simulink model "Medium_Self_Balance_Vehicle"  (R2021b)
settings: Solver=FixedStepDiscrete  StartTime=0.0  StopTime=10.0  FixedStep=0.005  RelTol=1e-3
libraries: TIMERS_Lib x9, GPIO_Lib x8, REG_Lib x4, ADC_Lib x1, STM32_Config_Lib x1, USART_Lib x1
(part 1 of 2)
settings Model: Creator=Administrator  LastModifiedBy=Li Chong
settings SolverCC: AlgebraicLoopSolver=TrustRegion
settings DataIOCC: ReturnWorkspaceOutputs=off
settings OptimizationCC: DefaultParameterBehavior=Inlined  EnhancedBackFolding=on  PassReuseOutputArgsAs=Individual arguments  OptimizeBlockOrder=speed  DifferentSizesBufferReuse=on  OptimizationCustomize=off  EfficientTunableParamExpr=on
settings DebuggingCC: AlgebraicLoopMsg=none  MultiTaskDSMMsg=none  ParameterPrecisionLossMsg=none  ParameterTunabilityLossMsg=error  SFMachineParentedDataDiag=warning  ArithmeticOperatorsInVariantConditions=warning
settings HardwareCC: ProdBitPerPointer=32  ProdBitPerSizeT=32  ProdBitPerPtrDiffT=32  ProdLargestAtomicInteger=Integer  ProdWordSize=32  ProdHWDeviceType=STMicroelectronics->STM32 32-bit Cortex-M
settings SFSimCC: SimCustomHeaderCode="#include \"myfile.h\""  SimUserSources=myfile.c  SimUseLocalCustomCode=off  MATLABDynamicMemAlloc=off  CustomCodeUndefinedFunction=UseInterfaceOnly
settings RTWCC: Description=stm32 (Embedded Target)  SystemTargetFile=stm32.tlc  TemplateMakefile=stm32.tmf  GenerateReport=on  RTWUseLocalCustomCode=off  CustomHeaderCode="#include \"delay.h\""  IncludeHyperlinkInReport=on  GenerateTraceInfo=on  GenerateTraceReport=on  GenerateTraceReportSl=on  GenerateTraceReportSf=on  GenerateTraceReportEml=on
settings CodeAppCC: ForceParamTrailComments=on  IgnoreCustomStorageClasses=off  MaxIdLength=64  OperatorAnnotations=on  SimulinkDataObjDesc=on  SFDataObjDesc=on  CustomSymbolStrType=$N$R$M  SimulinkBlockComments=off
settings STFCustomTargetCC: TargetLangStandard=C99 (ISO)  CodeReplacementLibrary=ARM CMSIS SIN COS  MultiwordLength=256  ParMdlRefBuildCompliant=on  IncludeMdlTerminateFcn=off  CombineOutputUpdateFcns=on  ERTCustomFileBanners=on  SupportContinuousTime=off  SupportNonInlinedSFcns=off  RemoveResetFunc=on  MATLABClassNameForMDSCustomization=Simulink.SoftwareTarget.ERTCustomization  GRTInterface=off  SystemTargetFile=stm32.tlc
settings ERTTargetCC: TargetLangStandard=C99 (ISO)  CodeReplacementLibrary=ARM CMSIS SIN COS  CompOptLevelCompliant=off  ConcurrentExecutionCompliant=off  IncludeMdlTerminateFcn=off  ModelStepFunctionPrototypeControlCompliant=off  CPPClassGenCompliant=off  UseToolchainInfoCompliant=off  ExtModeStaticAllocSize=256  ExtModeMexArgs=0,1,115200,10  InlinedParameterPlacement=NonHierarchical  ERTSrcFileBannerTemplate=sourceFileTemplate.cgt  ERTHdrFileBannerTemplate=sourceFileTemplate.cgt  ERTDataSrcFileTemplate=sourceFileTemplate.cgt  ERTDataHdrFileTemplate=sourceFileTemplate.cgt  ERTCustomFileTemplate=customRoutineProcess.tlc

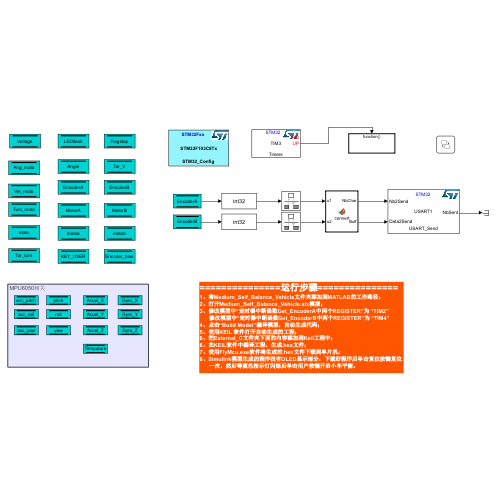
[thumbnail: Simulink's stored preview of the top-level diagram]
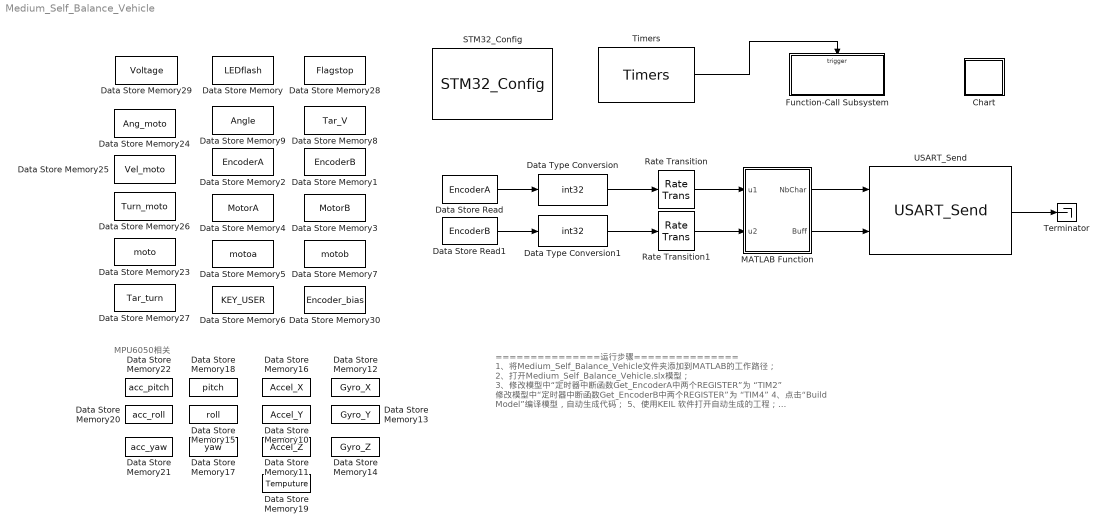
== system Medium_Self_Balance_Vehicle ==
  note: MPU6050相关
  note: ===============运行步骤===============
      | 1、将Medium_Self_Balance_Vehicle文件夹添加到MATLAB的工作路径；
      | 2、打开Medium_Self_Balance_Vehicle.slx模型；
      | 3、修改模型中“定时器中断函数Get_EncoderA中两个REGISTER”为 “TIM2”
      | 修改模型中“定时器中断函数Get_EncoderB中两个REGISTER”为 “TIM4”
      | 4、点击“Build Model”编译模型，自动生成代码；
      | 5、使用KEIL 软件打开自动生成的工程；
      | 6、把External_C文件夹下面的内容添加到Keil工程中；
      | 6、在KEIL软件中编译工程，生成.hex文件；
      | 7、使用FlyMcu.exe软件将生成的.hex文件下载到单片机；
      | 8、Simulink模型生成的程序没有OLED显示部分，下载好程序后单击复位按键复位 一次，然后等蓝色指示灯闪烁后单击用户按键开启小车平衡。
  Chart : Stateflow chart  Priority=1  TreatAsAtomicUnit=on
  Data Store Memory : DataStoreMemory  DataStoreName=LEDflash  ReadBeforeWriteMsg=warning  WriteAfterWriteMsg=warning  WriteAfterReadMsg=warning  ShowAdditionalParam=off
  Data Store Memory1 : DataStoreMemory  DataStoreName=EncoderB  ReadBeforeWriteMsg=warning  WriteAfterWriteMsg=warning  WriteAfterReadMsg=warning  ShowAdditionalParam=off  OutDataTypeStr=int16
  Data Store Memory10 : DataStoreMemory  DataStoreName=Accel_Y  ReadBeforeWriteMsg=warning  WriteAfterWriteMsg=warning  WriteAfterReadMsg=warning  ShowAdditionalParam=off  OutDataTypeStr=double
  Data Store Memory11 : DataStoreMemory  DataStoreName=Accel_Z  ReadBeforeWriteMsg=warning  WriteAfterWriteMsg=warning  WriteAfterReadMsg=warning  ShowAdditionalParam=off  OutDataTypeStr=double
  Data Store Memory12 : DataStoreMemory  DataStoreName=Gyro_X  ReadBeforeWriteMsg=warning  WriteAfterWriteMsg=warning  WriteAfterReadMsg=warning  ShowAdditionalParam=off  OutDataTypeStr=double
  Data Store Memory13 : DataStoreMemory  DataStoreName=Gyro_Y  ReadBeforeWriteMsg=warning  WriteAfterWriteMsg=warning  WriteAfterReadMsg=warning  ShowAdditionalParam=off  OutDataTypeStr=double
  Data Store Memory14 : DataStoreMemory  DataStoreName=Gyro_Z  ReadBeforeWriteMsg=warning  WriteAfterWriteMsg=warning  WriteAfterReadMsg=warning  ShowAdditionalParam=off  OutDataTypeStr=double
  Data Store Memory15 : DataStoreMemory  DataStoreName=roll  ReadBeforeWriteMsg=warning  WriteAfterWriteMsg=warning  WriteAfterReadMsg=warning  ShowAdditionalParam=off  OutDataTypeStr=double
  Data Store Memory16 : DataStoreMemory  DataStoreName=Accel_X  ReadBeforeWriteMsg=warning  WriteAfterWriteMsg=warning  WriteAfterReadMsg=warning  ShowAdditionalParam=off  OutDataTypeStr=double
  Data Store Memory17 : DataStoreMemory  DataStoreName=yaw  ReadBeforeWriteMsg=warning  WriteAfterWriteMsg=warning  WriteAfterReadMsg=warning  ShowAdditionalParam=off  OutDataTypeStr=double
  Data Store Memory18 : DataStoreMemory  DataStoreName=pitch  ReadBeforeWriteMsg=warning  WriteAfterWriteMsg=warning  WriteAfterReadMsg=warning  ShowAdditionalParam=off  OutDataTypeStr=double
  Data Store Memory19 : DataStoreMemory  DataStoreName=Temputure  ReadBeforeWriteMsg=warning  WriteAfterWriteMsg=warning  WriteAfterReadMsg=warning  ShowAdditionalParam=off  OutDataTypeStr=double
  Data Store Memory2 : DataStoreMemory  DataStoreName=EncoderA  ReadBeforeWriteMsg=warning  WriteAfterWriteMsg=warning  WriteAfterReadMsg=warning  ShowAdditionalParam=off  OutDataTypeStr=int16
  Data Store Memory20 : DataStoreMemory  DataStoreName=acc_roll  ReadBeforeWriteMsg=warning  WriteAfterWriteMsg=warning  WriteAfterReadMsg=warning  ShowAdditionalParam=off  OutDataTypeStr=double
  Data Store Memory21 : DataStoreMemory  DataStoreName=acc_yaw  ReadBeforeWriteMsg=warning  WriteAfterWriteMsg=warning  WriteAfterReadMsg=warning  ShowAdditionalParam=off  OutDataTypeStr=double
  Data Store Memory22 : DataStoreMemory  DataStoreName=acc_pitch  ReadBeforeWriteMsg=warning  WriteAfterWriteMsg=warning  WriteAfterReadMsg=warning  ShowAdditionalParam=off  OutDataTypeStr=double
  Data Store Memory23 : DataStoreMemory  DataStoreName=moto  ReadBeforeWriteMsg=warning  WriteAfterWriteMsg=warning  WriteAfterReadMsg=warning  ShowAdditionalParam=off
  Data Store Memory24 : DataStoreMemory  DataStoreName=Ang_moto  ReadBeforeWriteMsg=warning  WriteAfterWriteMsg=warning  WriteAfterReadMsg=warning  ShowAdditionalParam=off
  Data Store Memory25 : DataStoreMemory  DataStoreName=Vel_moto  ReadBeforeWriteMsg=warning  WriteAfterWriteMsg=warning  WriteAfterReadMsg=warning  ShowAdditionalParam=off
  Data Store Memory26 : DataStoreMemory  DataStoreName=Turn_moto  ReadBeforeWriteMsg=warning  WriteAfterWriteMsg=warning  WriteAfterReadMsg=warning  ShowAdditionalParam=off
  Data Store Memory27 : DataStoreMemory  DataStoreName=Tar_turn  ReadBeforeWriteMsg=warning  WriteAfterWriteMsg=warning  WriteAfterReadMsg=warning  ShowAdditionalParam=off
  Data Store Memory28 : DataStoreMemory  DataStoreName=Flagstop  ReadBeforeWriteMsg=warning  WriteAfterWriteMsg=warning  WriteAfterReadMsg=warning  InitialValue=1  ShowAdditionalParam=off  OutDataTypeStr=boolean
  Data Store Memory29 : DataStoreMemory  DataStoreName=Voltage  ReadBeforeWriteMsg=warning  WriteAfterWriteMsg=warning  WriteAfterReadMsg=warning  ShowAdditionalParam=off  OutDataTypeStr=double
  Data Store Memory3 : DataStoreMemory  DataStoreName=MotorB  ReadBeforeWriteMsg=warning  WriteAfterWriteMsg=warning  WriteAfterReadMsg=warning  ShowAdditionalParam=off  OutDataTypeStr=double
  Data Store Memory30 : DataStoreMemory  DataStoreName=Encoder_bias  ReadBeforeWriteMsg=warning  WriteAfterWriteMsg=warning  WriteAfterReadMsg=warning  ShowAdditionalParam=off  OutDataTypeStr=double
  Data Store Memory4 : DataStoreMemory  DataStoreName=MotorA  ReadBeforeWriteMsg=warning  WriteAfterWriteMsg=warning  WriteAfterReadMsg=warning  ShowAdditionalParam=off  OutDataTypeStr=double
  Data Store Memory5 : DataStoreMemory  DataStoreName=motoa  ReadBeforeWriteMsg=warning  WriteAfterWriteMsg=warning  WriteAfterReadMsg=warning  ShowAdditionalParam=off  OutDataTypeStr=int16
  Data Store Memory6 : DataStoreMemory  DataStoreName=KEY_USER  ReadBeforeWriteMsg=warning  WriteAfterWriteMsg=warning  WriteAfterReadMsg=warning  ShowAdditionalParam=off  OutDataTypeStr=int16
  Data Store Memory7 : DataStoreMemory  DataStoreName=motob  ReadBeforeWriteMsg=warning  WriteAfterWriteMsg=warning  WriteAfterReadMsg=warning  ShowAdditionalParam=off  OutDataTypeStr=int16
  Data Store Memory8 : DataStoreMemory  DataStoreName=Tar_V  ReadBeforeWriteMsg=warning  WriteAfterWriteMsg=warning  WriteAfterReadMsg=warning  ShowAdditionalParam=off  OutDataTypeStr=int16
  Data Store Memory9 : DataStoreMemory  DataStoreName=Angle  ReadBeforeWriteMsg=warning  WriteAfterWriteMsg=warning  WriteAfterReadMsg=warning  ShowAdditionalParam=off  OutDataTypeStr=double
  Data Store Read : DataStoreRead  DataStoreName=EncoderA  SampleTime=0.05  IndexOptions=Index vector (dialog)  Indices=1  OutputSizes=1
  Data Store Read1 : DataStoreRead  DataStoreName=EncoderB  SampleTime=0.05  IndexOptions=Index vector (dialog)  Indices=1  OutputSizes=1
  Data Type Conversion : DataTypeConversion  OutDataTypeStr=int32
  Data Type Conversion1 : DataTypeConversion  OutDataTypeStr=int32
  Function-Call Subsystem : Subsystem  TreatAsAtomicUnit=on
  MATLAB Function : MATLAB Function  TreatAsAtomicUnit=on
  Rate Transition : RateTransition  OutPortSampleTimeMultiple=10  OutPortSampleTime=0.05
  Rate Transition1 : RateTransition  OutPortSampleTimeMultiple=10  OutPortSampleTime=0.05
  STM32_Config : STM32_Config_Lib/STM32_Config  Priority=0  Project_Path=.\  Config_File=Medium_Self_Balance_Vehicle.ioc  MCU_Name=STM32F103C8Tx
      settings: SourceProductName=Target Support Package - STM32 Adapter
  Terminator : Terminator
  Timers : TIMERS_Lib/Timers  Priority=2  currentTIM=TIM3  TIM_Name=TIM3  sysUsingTimer=off  TIM_APBClock=72000000  TIM_Set_Clk=off  TIM_Prescaler=7199  TIM_Clock=10000.00  Variable_frequency=off  TIM_Set_OutFreq=off  TIM_ARR=49  Output_frequency=204.08  Repetition_counter=0  TIM_Mode=Up  TIM_DMA=none  TIM_IRQ=on  TIM_IRQ_ONLY=on  TIM_UP=on  TIM_TRG=off  TIM_COM=off  TIM_BRK=off  NbTIM=4  CH1_enable=off  CH1N_enable=off  CH1_type=Unknown  CH1_DMA=off  CH1_int=off  CH1_edge=Rising  CH1_div=1  CH1_variable_duty=off  CH1_set_pulse=off  CH1_output_duty=0.00  CH1_pulse=0  CH2_enable=off  CH2N_enable=off  CH2_type=Unknown  CH2_DMA=off  CH2_int=off  CH2_edge=Rising  CH2_div=1  CH2_variable_duty=off  CH2_set_pulse=off  CH2_output_duty=0.00  CH2_pulse=0  CH3_enable=off  CH3N_enable=off  CH3_type=Unknown  CH3_DMA=off  CH3_int=off  CH3_edge=Rising  CH3_div=1  CH3_variable_duty=off  CH3_set_pulse=off  CH3_output_duty=0.00  CH3_pulse=0  CH4_enable=off  CH4N_enable=off  CH4_type=Unknown  CH4_DMA=off  CH4_int=off  CH4_edge=Rising  CH4_div=1  CH4_variable_duty=off  CH4_set_pulse=off  CH4_output_duty=0.00  CH4_pulse=0
      settings: SourceProductName=Target Support Package - STM32 Adapter
  USART_Send : USART_Lib/USART_Send  USART_name=USART1  Buff_size=56  nbUsart=1  usartMode=Asynchronous  usartDma_Rx=off  usartDma_Tx=off  usartIt=on
      settings: SourceProductName=Target Support Package - STM32 Adapter
  wires:
  MATLAB Function/1(NbChar) -> USART_Send/1
  Data Store Read/1 -> Data Type Conversion/1
  USART_Send/1 -> Terminator/1
  MATLAB Function/2(Buff) -> USART_Send/2
  Data Store Read1/1 -> Data Type Conversion1/1
  Timers/1 -> Function-Call Subsystem/Trigger
  Data Type Conversion1/1 -> Rate Transition1/1
  Data Type Conversion/1 -> Rate Transition/1
  Rate Transition1/1 -> MATLAB Function/2(u2)
  Rate Transition/1 -> MATLAB Function/1(u1)

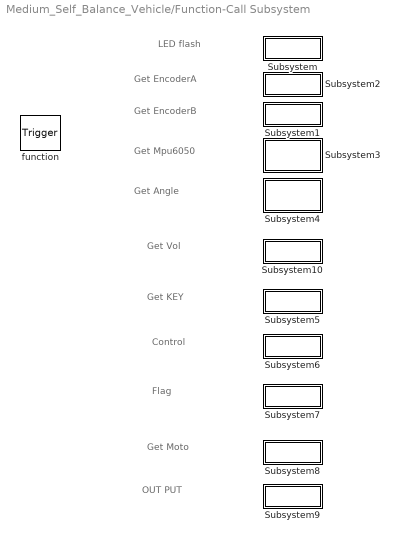
== system Medium_Self_Balance_Vehicle/Function-Call Subsystem ==
  note: Get Moto
  note: Get EncoderA
  note: OUT PUT
  note: LED flash
  note: Get KEY
  note: Get EncoderB
  note: Get Mpu6050
  note: Get Angle
  note: Control
  note: Flag
  note: Get Vol
  function : TriggerPort  TriggerType=function-call  VariantControl=Variant
  Subsystem : Subsystem  Priority=0
  Subsystem1 : Subsystem  Priority=1
  Subsystem10 : Subsystem  Priority=4
  Subsystem2 : Subsystem  Priority=1
  Subsystem3 : Subsystem  Priority=2
  Subsystem4 : Subsystem  Priority=3
  Subsystem5 : Subsystem  Priority=5
  Subsystem6 : Subsystem  Priority=6
  Subsystem7 : Subsystem  Priority=7
  Subsystem8 : Subsystem  Priority=8
  Subsystem9 : Subsystem  Priority=9

== system Medium_Self_Balance_Vehicle/Function-Call Subsystem/Subsystem ==
  Add : Sum
  Constant : Constant
  Data Store Read1 : DataStoreRead  DataStoreName=LEDflash  IndexOptions=Index vector (dialog)  Indices=1  OutputSizes=1
  Data Store Write : DataStoreWrite  DataStoreName=LEDflash  IndexOptions=Index vector (dialog)  Indices=1  OutputSizes=1
  If : If  IfExpression=u1 > 200
  If Action Subsystem : Subsystem  TreatAsAtomicUnit=on
  Terminator : Terminator
  wires:
  Constant/1 -> Add/2
  If/1 -> If Action Subsystem/Action
  If/2 -> Terminator/1
  Add/1 -> Data Store Write/1, If/1
  Data Store Read1/1 -> Add/1

== system Medium_Self_Balance_Vehicle/Function-Call Subsystem/Subsystem1 ==
  Data Store Write1 : DataStoreWrite  Priority=2  DataStoreName=EncoderB  IndexOptions=Index vector (dialog)  Indices=1  OutputSizes=1
  REG_Access2 : REG_Lib/REG_Access  Priority=2  Peripheral=ADC1  RegName=CNT  RegRead=off  RegWrite=on  RegValueIn=off  RegValue=0  RegEqual=on  RegAnd=off  RegOr=off  RegComplement=off  currentPeriph=ADC1
      settings: SourceProductName=Target Support Package - STM32 Adapter
  REG_Access3 : REG_Lib/REG_Access  Priority=1  Peripheral=ADC1  RegName=CNT  RegRead=on  RegWrite=off  RegValueIn=off  RegValue=0  RegEqual=on  RegAnd=off  RegOr=off  RegComplement=off  currentPeriph=ADC1
      settings: SourceProductName=Target Support Package - STM32 Adapter
  Timers1 : TIMERS_Lib/Timers  currentTIM=TIM4  TIM_Name=TIM4  sysUsingTimer=off  TIM_APBClock=72000000  TIM_Set_Clk=off  TIM_Prescaler=0  TIM_Clock=72000000.00  Variable_frequency=off  TIM_Set_OutFreq=off  TIM_ARR=65536  Output_frequency=1098.63  Repetition_counter=0  TIM_Mode=Up  TIM_DMA=none  TIM_IRQ=on  TIM_IRQ_ONLY=on  TIM_UP=off  TIM_TRG=off  TIM_COM=off  TIM_BRK=off  NbTIM=4  CH1_enable=on  CH1N_enable=off  CH1_type=Input_Encoder  CH1_DMA=off  CH1_int=off  CH1_edge=Rising  CH1_div=1  CH1_variable_duty=off  CH1_set_pulse=off  CH1_output_duty=0.00  CH1_pulse=0  CH2_enable=on  CH2N_enable=off  CH2_type=Input_Encoder  CH2_DMA=off  CH2_int=off  CH2_edge=Rising  CH2_div=1  CH2_variable_duty=off  CH2_set_pulse=off  CH2_output_duty=0.00  CH2_pulse=0  CH3_enable=off  CH3N_enable=off  CH3_type=Unknown  CH3_DMA=off  CH3_int=off  CH3_edge=Rising  CH3_div=1  CH3_variable_duty=off  CH3_set_pulse=off  CH3_output_duty=0.00  CH3_pulse=0  CH4_enable=off  CH4N_enable=off  CH4_type=Unknown  CH4_DMA=off  CH4_int=off  CH4_edge=Rising  CH4_div=1  CH4_variable_duty=off  CH4_set_pulse=off  CH4_output_duty=0.00  CH4_pulse=0
      settings: SourceProductName=Target Support Package - STM32 Adapter
  wires:
  REG_Access3/1 -> Data Store Write1/1

== system Medium_Self_Balance_Vehicle/Function-Call Subsystem/Subsystem10 ==
  1/10 : Gain  Gain=0.1
  3.3*11/4096 : Gain  Gain=0.00886
  ADC_Read : ADC_Lib/ADC_Read  Priority=1  ADC_Name=ADC1  ADC_Ch0=off  ADC_Ch1=off  ADC_Ch2=off  ADC_Ch3=off  ADC_Ch4=off  ADC_Ch5=off  ADC_Ch6=on  ADC_Ch7=off  ADC_Ch8=off  ADC_Ch9=off  ADC_Ch10=off  ADC_Ch11=off  ADC_Ch12=off  ADC_Ch13=off  ADC_Ch14=off  ADC_Ch15=off  ADC_Ch16=off  ADC_Ch17=off  ADC_Ch18=off  RgRk1=on  RgRk2=off  RgRk3=off  RgRk4=off  RgRk1_Ch=Ch6_r1  RgRk2_Ch=off  RgRk3_Ch=off  RgRk4_Ch=off  RgRk5=off  RgRk6=off  RgRk7=off  RgRk8=off  RgRk5_Ch=off  RgRk6_Ch=off  RgRk7_Ch=off  RgRk8_Ch=off  RgRk9=off  RgRk10=off  RgRk11=off  RgRk12=off  RgRk9_Ch=off  RgRk10_Ch=off  RgRk11_Ch=off  RgRk12_Ch=off  RgRk13=off  RgRk14=off  RgRk15=off  RgRk16=off  RgRk13_Ch=off  RgRk14_Ch=off  RgRk15_Ch=off  RgRk16_Ch=off  InjRk1=off  InjRk2=off  InjRk3=off  InjRk4=off  InjRk1_Ch=off  InjRk2_Ch=off  InjRk3_Ch=off  InjRk4_Ch=off  ADC_Trig=Not used  ADC_TrigEdge=Not used  DmaReq=off  DMA_Buffer=0  ItReq=off  AWD_Mode=NOT_USED  AWD_Ch=0  AWD_HThres=0  AWD_LThres=0  AWD_En_Int=off  AWD2_HThres=0  AWD2_LThres=0  AWD2_En_Int=off  AWD3_HThres=0  AWD3_LThres=0  AWD3_En_Int=off  EOC_SEQ=off  EOC_IT=off  JEOC_IT=off  AWD_IT=off  OVR_IT=off  CpltTrans=off  HalfTrans=off  ADC_RegNb=1  ADC_RegCh0=off  ADC_RegCh1=off  ADC_RegCh2=off  ADC_RegCh3=off  ADC_RegCh4=off  ADC_RegCh5=off  ADC_RegCh6=on  ADC_RegCh7=off  ADC_RegCh8=off  ADC_RegCh9=off  ADC_RegCh10=off  ADC_RegCh11=off  ADC_RegCh12=off  ADC_RegCh13=off  ADC_RegCh14=off  ADC_RegCh15=off  ADC_RegCh16=off  ADC_RegCh17=off  ADC_RegCh18=off  ADC_InjNb=0  ADC_InjCh0=off  ADC_InjCh1=off  ADC_InjCh2=off  ADC_InjCh3=off  ADC_InjCh4=off  ADC_InjCh5=off  ADC_InjCh6=off  ADC_InjCh7=off  ADC_InjCh8=off  ADC_InjCh9=off  ADC_InjCh10=off  ADC_InjCh11=off  ADC_InjCh12=off  ADC_InjCh13=off  ADC_InjCh14=off  ADC_InjCh15=off  ADC_InjCh16=off  ADC_InjCh17=off  ADC_InjCh18=off  NbADC=1  CurrentADC=ADC1
      settings: SourceProductName=Target Support Package - STM32 Adapter
  Data Store Write : DataStoreWrite  DataStoreName=Voltage  IndexOptions=Index vector (dialog)  Indices=1  OutputSizes=1
  For Iterator Subsystem1 : Subsystem  Priority=4  TreatAsAtomicUnit=on
  wires:
  For Iterator Subsystem1/1(Out1) -> 1/10/1
  1/10/1 -> 3.3*11/4096/1
  3.3*11/4096/1 -> Data Store Write/1
  ADC_Read/1 -> For Iterator Subsystem1/1(In1)

== system Medium_Self_Balance_Vehicle/Function-Call Subsystem/Subsystem2 ==
  Data Store Write4 : DataStoreWrite  Priority=2  DataStoreName=EncoderA  IndexOptions=Index vector (dialog)  Indices=1  OutputSizes=1
  REG_Access : REG_Lib/REG_Access  Priority=2  Peripheral=ADC1  RegName=CNT  RegRead=off  RegWrite=on  RegValueIn=off  RegValue=0  RegEqual=on  RegAnd=off  RegOr=off  RegComplement=off  currentPeriph=ADC1
      settings: SourceProductName=Target Support Package - STM32 Adapter
  REG_Access1 : REG_Lib/REG_Access  Priority=1  Peripheral=ADC1  RegName=CNT  RegRead=on  RegWrite=off  RegValueIn=off  RegValue=0  RegEqual=on  RegAnd=off  RegOr=off  RegComplement=off  currentPeriph=ADC1
      settings: SourceProductName=Target Support Package - STM32 Adapter
  Timers : TIMERS_Lib/Timers  currentTIM=TIM2  TIM_Name=TIM2  sysUsingTimer=off  TIM_APBClock=72000000  TIM_Set_Clk=off  TIM_Prescaler=0  TIM_Clock=72000000.00  Variable_frequency=off  TIM_Set_OutFreq=off  TIM_ARR=65536  Output_frequency=1098.63  Repetition_counter=0  TIM_Mode=Up  TIM_DMA=none  TIM_IRQ=on  TIM_IRQ_ONLY=on  TIM_UP=off  TIM_TRG=off  TIM_COM=off  TIM_BRK=off  NbTIM=4  CH1_enable=on  CH1N_enable=off  CH1_type=Input_Encoder  CH1_DMA=off  CH1_int=off  CH1_edge=Rising  CH1_div=1  CH1_variable_duty=off  CH1_set_pulse=off  CH1_output_duty=0.00  CH1_pulse=0  CH2_enable=on  CH2N_enable=off  CH2_type=Input_Encoder  CH2_DMA=off  CH2_int=off  CH2_edge=Rising  CH2_div=1  CH2_variable_duty=off  CH2_set_pulse=off  CH2_output_duty=0.00  CH2_pulse=0  CH3_enable=off  CH3N_enable=off  CH3_type=Unknown  CH3_DMA=off  CH3_int=off  CH3_edge=Rising  CH3_div=1  CH3_variable_duty=off  CH3_set_pulse=off  CH3_output_duty=0.00  CH3_pulse=0  CH4_enable=off  CH4N_enable=off  CH4_type=Unknown  CH4_DMA=off  CH4_int=off  CH4_edge=Rising  CH4_div=1  CH4_variable_duty=off  CH4_set_pulse=off  CH4_output_duty=0.00  CH4_pulse=0
      settings: SourceProductName=Target Support Package - STM32 Adapter
  wires:
  REG_Access1/1 -> Data Store Write4/1

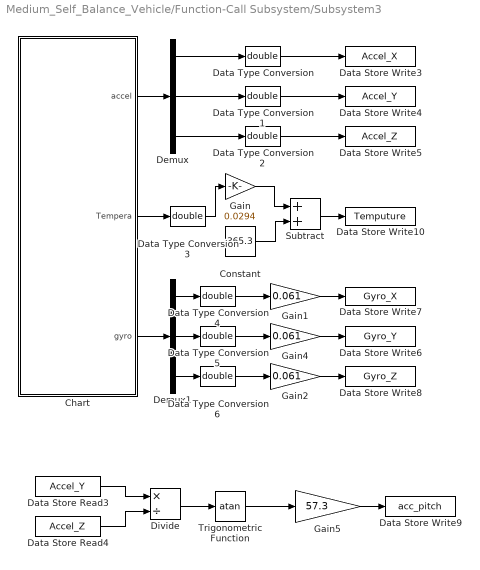
== system Medium_Self_Balance_Vehicle/Function-Call Subsystem/Subsystem3 ==
  Chart : Stateflow chart  TreatAsAtomicUnit=on
  Constant : Constant  Value=365.3  OutDataTypeStr=double
  Data Store Read3 : DataStoreRead  DataStoreName=Accel_Y  IndexOptions=Index vector (dialog)  Indices=1  OutputSizes=1
  Data Store Read4 : DataStoreRead  DataStoreName=Accel_Z  IndexOptions=Index vector (dialog)  Indices=1  OutputSizes=1
  Data Store Write10 : DataStoreWrite  DataStoreName=Temputure  IndexOptions=Index vector (dialog)  Indices=1  OutputSizes=1
  Data Store Write3 : DataStoreWrite  DataStoreName=Accel_X  IndexOptions=Index vector (dialog)  Indices=1  OutputSizes=1
  Data Store Write4 : DataStoreWrite  DataStoreName=Accel_Y  IndexOptions=Index vector (dialog)  Indices=1  OutputSizes=1
  Data Store Write5 : DataStoreWrite  DataStoreName=Accel_Z  IndexOptions=Index vector (dialog)  Indices=1  OutputSizes=1
  Data Store Write6 : DataStoreWrite  DataStoreName=Gyro_Y  IndexOptions=Index vector (dialog)  Indices=1  OutputSizes=1
  Data Store Write7 : DataStoreWrite  DataStoreName=Gyro_X  IndexOptions=Index vector (dialog)  Indices=1  OutputSizes=1
  Data Store Write8 : DataStoreWrite  DataStoreName=Gyro_Z  IndexOptions=Index vector (dialog)  Indices=1  OutputSizes=1
  Data Store Write9 : DataStoreWrite  DataStoreName=acc_pitch  IndexOptions=Index vector (dialog)  Indices=1  OutputSizes=1
  Data Type Conversion{,1..6} (7 alike) : DataTypeConversion  OutDataTypeStr=double
  Demux : Demux  Outputs=3
  Demux1 : Demux  Outputs=3
  Divide : Product  Inputs=*/
  Gain : Gain  Gain=0.0294  OutDataTypeStr=double
  Gain1 : Gain  Gain=0.061  OutDataTypeStr=double
  Gain2 : Gain  Gain=0.061  OutDataTypeStr=double
  Gain4 : Gain  Gain=0.061  OutDataTypeStr=double
  Gain5 : Gain  Gain=57.3  OutDataTypeStr=double
  Subtract : Sum  OutDataTypeStr=double
  Trigonometric Function : Trigonometry  Operator=atan
  wires:
  Demux/2 -> Data Type Conversion1/1
  Demux/1 -> Data Type Conversion/1
  Demux/3 -> Data Type Conversion2/1
  Demux1/2 -> Data Type Conversion5/1
  Demux1/3 -> Data Type Conversion6/1
  Demux1/1 -> Data Type Conversion4/1
  Chart/3(gyro) -> Demux1/1
  Chart/1(accel) -> Demux/1
  Gain/1 -> Subtract/1
  Constant/1 -> Subtract/2
  Subtract/1 -> Data Store Write10/1
  Gain1/1 -> Data Store Write7/1
  Gain4/1 -> Data Store Write6/1
  Gain2/1 -> Data Store Write8/1
  Data Type Conversion/1 -> Data Store Write3/1
  Data Type Conversion1/1 -> Data Store Write4/1
  Data Type Conversion2/1 -> Data Store Write5/1
  Chart/2(Tempera) -> Data Type Conversion3/1
  Data Type Conversion3/1 -> Gain/1
  Data Type Conversion4/1 -> Gain1/1
  Data Type Conversion6/1 -> Gain2/1
  Data Type Conversion5/1 -> Gain4/1
  Data Store Read4/1 -> Divide/2
  Data Store Read3/1 -> Divide/1
  Divide/1 -> Trigonometric Function/1
  Gain5/1 -> Data Store Write9/1
  Trigonometric Function/1 -> Gain5/1

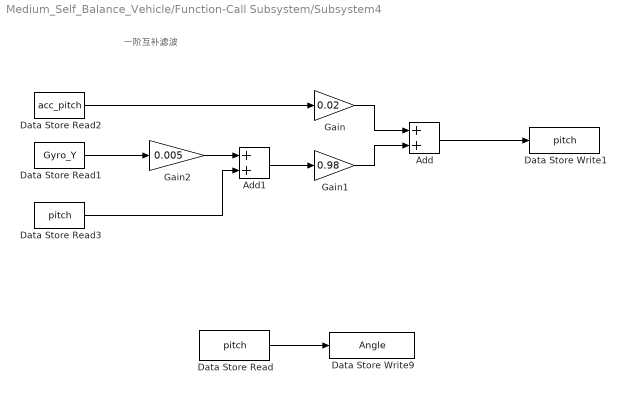
== system Medium_Self_Balance_Vehicle/Function-Call Subsystem/Subsystem4 ==
  note: 一阶互补滤波
  Add : Sum
  Add1 : Sum
  Data Store Read : DataStoreRead  DataStoreName=pitch  IndexOptions=Index vector (dialog)  Indices=1  OutputSizes=1
  Data Store Read1 : DataStoreRead  DataStoreName=Gyro_Y  IndexOptions=Index vector (dialog)  Indices=1  OutputSizes=1
  Data Store Read2 : DataStoreRead  DataStoreName=acc_pitch  IndexOptions=Index vector (dialog)  Indices=1  OutputSizes=1
  Data Store Read3 : DataStoreRead  DataStoreName=pitch  IndexOptions=Index vector (dialog)  Indices=1  OutputSizes=1
  Data Store Write1 : DataStoreWrite  DataStoreName=pitch  IndexOptions=Index vector (dialog)  Indices=1  OutputSizes=1
  Data Store Write9 : DataStoreWrite  DataStoreName=Angle  IndexOptions=Index vector (dialog)  Indices=1  OutputSizes=1
  Gain : Gain  Gain=0.02
  Gain1 : Gain  Gain=0.98
  Gain2 : Gain  Gain=0.005
  wires:
  Data Store Read/1 -> Data Store Write9/1
  Add1/1 -> Gain1/1
  Add/1 -> Data Store Write1/1
  Gain1/1 -> Add/2
  Data Store Read1/1 -> Gain2/1
  Data Store Read2/1 -> Gain/1
  Gain/1 -> Add/1
  Gain2/1 -> Add1/1
  Data Store Read3/1 -> Add1/2

== system Medium_Self_Balance_Vehicle/Function-Call Subsystem/Subsystem5 ==
  Atomic Subsystem : Subsystem  TreatAsAtomicUnit=on
  Data Store Read : DataStoreRead  DataStoreName=KEY_USER  IndexOptions=Index vector (dialog)  Indices=1  OutputSizes=1
  Data Store Write : DataStoreWrite  DataStoreName=KEY_USER  IndexOptions=Index vector (dialog)  Indices=1  OutputSizes=1
  GPIO_Read : GPIO_Lib/GPIO_Read  Port_name=GPIOA  Pin_0=off  Pin_1=off  Pin_2=off  Pin_3=off  Pin_4=off  Pin_5=on  Pin_6=off  Pin_7=off  Pin_8=off  Pin_9=off  Pin_10=off  Pin_11=off  Pin_12=off  Pin_13=off  Pin_14=off  Pin_15=off  PinList=GPIOA5
      settings: SourceProductName=Target Support Package - STM32 Adapter
  If : If  IfExpression=u1 == 1
  If Action Subsystem : Subsystem  TreatAsAtomicUnit=on
  Terminator : Terminator
  wires:
  Atomic Subsystem/1(Out1) -> Data Store Write/1
  GPIO_Read/1 -> Atomic Subsystem/1(In1)
  Data Store Read/1 -> If/1
  If/2 -> Terminator/1
  If/1 -> If Action Subsystem/Action

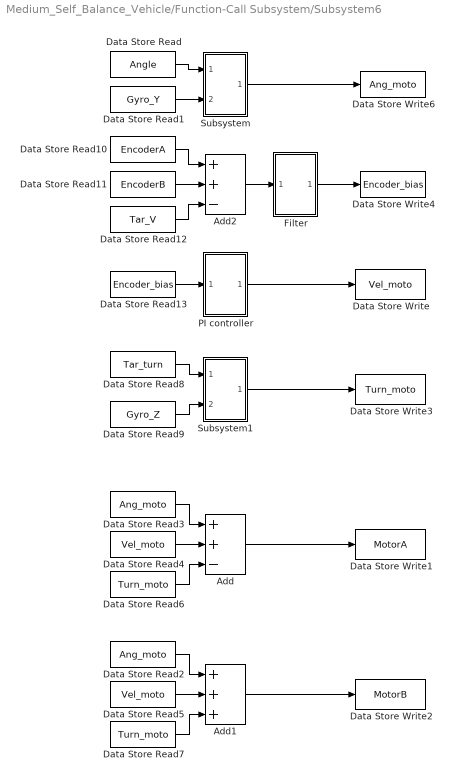
== system Medium_Self_Balance_Vehicle/Function-Call Subsystem/Subsystem6 ==
  Add : Sum  Priority=5  Inputs=++-
  Add1 : Sum  Priority=6  Inputs=+++
  Add2 : Sum  Priority=2  Inputs=++-
  Data Store Read : DataStoreRead  DataStoreName=Angle  IndexOptions=Index vector (dialog)  Indices=1  OutputSizes=1
  Data Store Read1 : DataStoreRead  DataStoreName=Gyro_Y  IndexOptions=Index vector (dialog)  Indices=1  OutputSizes=1
  Data Store Read10 : DataStoreRead  DataStoreName=EncoderA  IndexOptions=Index vector (dialog)  Indices=1  OutputSizes=1
  Data Store Read11 : DataStoreRead  DataStoreName=EncoderB  IndexOptions=Index vector (dialog)  Indices=1  OutputSizes=1
  Data Store Read12 : DataStoreRead  DataStoreName=Tar_V  IndexOptions=Index vector (dialog)  Indices=1  OutputSizes=1
  Data Store Read13 : DataStoreRead  DataStoreName=Encoder_bias  IndexOptions=Index vector (dialog)  Indices=1  OutputSizes=1
  Data Store Read2 : DataStoreRead  DataStoreName=Ang_moto  IndexOptions=Index vector (dialog)  Indices=1  OutputSizes=1
  Data Store Read3 : DataStoreRead  DataStoreName=Ang_moto  IndexOptions=Index vector (dialog)  Indices=1  OutputSizes=1
  Data Store Read4 : DataStoreRead  DataStoreName=Vel_moto  IndexOptions=Index vector (dialog)  Indices=1  OutputSizes=1
  Data Store Read5 : DataStoreRead  DataStoreName=Vel_moto  IndexOptions=Index vector (dialog)  Indices=1  OutputSizes=1
  Data Store Read6 : DataStoreRead  DataStoreName=Turn_moto  IndexOptions=Index vector (dialog)  Indices=1  OutputSizes=1
  Data Store Read7 : DataStoreRead  DataStoreName=Turn_moto  IndexOptions=Index vector (dialog)  Indices=1  OutputSizes=1
  Data Store Read8 : DataStoreRead  DataStoreName=Tar_turn  IndexOptions=Index vector (dialog)  Indices=1  OutputSizes=1
  Data Store Read9 : DataStoreRead  DataStoreName=Gyro_Z  IndexOptions=Index vector (dialog)  Indices=1  OutputSizes=1
  Data Store Write : DataStoreWrite  DataStoreName=Vel_moto  IndexOptions=Index vector (dialog)  Indices=1  OutputSizes=1
  Data Store Write1 : DataStoreWrite  DataStoreName=MotorA  IndexOptions=Index vector (dialog)  Indices=1  OutputSizes=1
  Data Store Write2 : DataStoreWrite  DataStoreName=MotorB  IndexOptions=Index vector (dialog)  Indices=1  OutputSizes=1
  Data Store Write3 : DataStoreWrite  DataStoreName=Turn_moto  IndexOptions=Index vector (dialog)  Indices=1  OutputSizes=1
  Data Store Write4 : DataStoreWrite  DataStoreName=Encoder_bias  IndexOptions=Index vector (dialog)  Indices=1  OutputSizes=1
  Data Store Write6 : DataStoreWrite  DataStoreName=Ang_moto  IndexOptions=Index vector (dialog)  Indices=1  OutputSizes=1
  Filter : Subsystem
  PI controller : Subsystem  Priority=3
  Subsystem : Subsystem  Priority=1
  Subsystem1 : Subsystem  Priority=4
  wires:
  Data Store Read/1 -> Subsystem/1(In1)
  Data Store Read1/1 -> Subsystem/2(In2)
  Subsystem/1(Out1) -> Data Store Write6/1
  Data Store Read3/1 -> Add/1
  Data Store Read4/1 -> Add/2
  Add/1 -> Data Store Write1/1
  Data Store Read6/1 -> Add/3
  Add1/1 -> Data Store Write2/1
  Data Store Read7/1 -> Add1/3
  Data Store Read5/1 -> Add1/2
  Data Store Read2/1 -> Add1/1
  Data Store Read8/1 -> Subsystem1/1(In1)
  Data Store Read9/1 -> Subsystem1/2(In2)
  Subsystem1/1(Out1) -> Data Store Write3/1
  Add2/1 -> Filter/1(In1)
  Data Store Read10/1 -> Add2/1
  Data Store Read11/1 -> Add2/2
  Data Store Read12/1 -> Add2/3
  Filter/1(Out1) -> Data Store Write4/1
  Data Store Read13/1 -> PI controller/1(In1)
  PI controller/1(Out1) -> Data Store Write/1

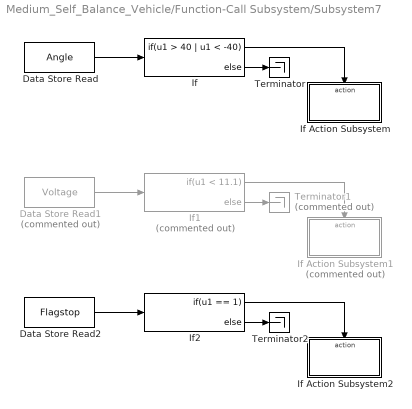
== system Medium_Self_Balance_Vehicle/Function-Call Subsystem/Subsystem7 ==
  Data Store Read : DataStoreRead  DataStoreName=Angle  IndexOptions=Index vector (dialog)  Indices=1  OutputSizes=1
  Data Store Read1 : DataStoreRead  Commented=on  DataStoreName=Voltage  IndexOptions=Index vector (dialog)  Indices=1  OutputSizes=1
  Data Store Read2 : DataStoreRead  DataStoreName=Flagstop  IndexOptions=Index vector (dialog)  Indices=1  OutputSizes=1
  If : If  IfExpression=u1 > 40 | u1 < -40
  If Action Subsystem : Subsystem  TreatAsAtomicUnit=on
  If Action Subsystem1 : Subsystem  Commented=on  TreatAsAtomicUnit=on
  If Action Subsystem2 : Subsystem  TreatAsAtomicUnit=on
  If1 : If  Commented=on  IfExpression=u1 < 11.1
  If2 : If  IfExpression=u1 == 1
  Terminator : Terminator
  Terminator1 : Terminator  Commented=on
  Terminator2 : Terminator
  wires:
  Data Store Read/1 -> If/1
  If/1 -> If Action Subsystem/Action
  If/2 -> Terminator/1
  If1/1 -> If Action Subsystem1/Action
  Data Store Read1/1 -> If1/1
  If1/2 -> Terminator1/1
  Data Store Read2/1 -> If2/1
  If2/2 -> Terminator2/1
  If2/1 -> If Action Subsystem2/Action

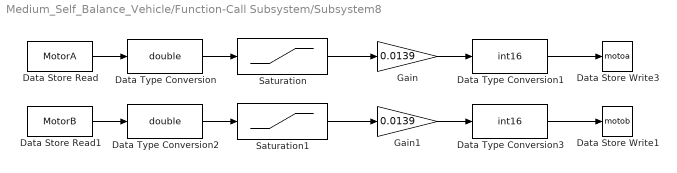
== system Medium_Self_Balance_Vehicle/Function-Call Subsystem/Subsystem8 ==
  Data Store Read : DataStoreRead  DataStoreName=MotorA  IndexOptions=Index vector (dialog)  Indices=1  OutputSizes=1
  Data Store Read1 : DataStoreRead  DataStoreName=MotorB  IndexOptions=Index vector (dialog)  Indices=1  OutputSizes=1
  Data Store Write1 : DataStoreWrite  DataStoreName=motob  IndexOptions=Index vector (dialog)  Indices=1  OutputSizes=1
  Data Store Write3 : DataStoreWrite  DataStoreName=motoa  IndexOptions=Index vector (dialog)  Indices=1  OutputSizes=1
  Data Type Conversion : DataTypeConversion  OutDataTypeStr=double
  Data Type Conversion1 : DataTypeConversion  OutDataTypeStr=int16
  Data Type Conversion2 : DataTypeConversion  OutDataTypeStr=double
  Data Type Conversion3 : DataTypeConversion  OutDataTypeStr=int16
  Gain : Gain  Gain=0.0139
  Gain1 : Gain  Gain=0.0139
  Saturation : Saturate  UpperLimit=6900  LowerLimit=-6900
  Saturation1 : Saturate  UpperLimit=6900  LowerLimit=-6900
  wires:
  Saturation/1 -> Gain/1
  Data Store Read/1 -> Data Type Conversion/1
  Gain/1 -> Data Type Conversion1/1
  Data Type Conversion/1 -> Saturation/1
  Data Type Conversion1/1 -> Data Store Write3/1
  Data Type Conversion2/1 -> Saturation1/1
  Gain1/1 -> Data Type Conversion3/1
  Data Store Read1/1 -> Data Type Conversion2/1
  Data Type Conversion3/1 -> Data Store Write1/1
  Saturation1/1 -> Gain1/1

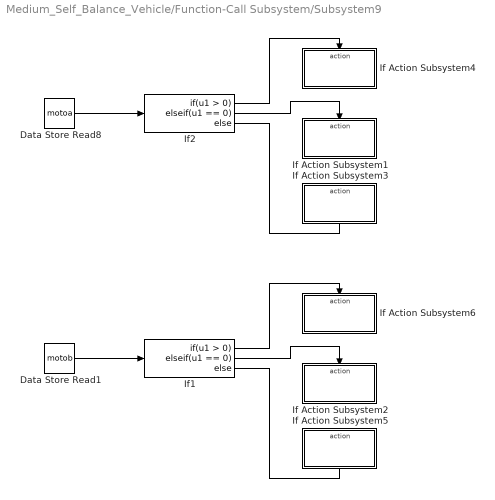
== system Medium_Self_Balance_Vehicle/Function-Call Subsystem/Subsystem9 ==
  Data Store Read1 : DataStoreRead  DataStoreName=motob  IndexOptions=Index vector (dialog)  Indices=1  OutputSizes=1
  Data Store Read8 : DataStoreRead  DataStoreName=motoa  IndexOptions=Index vector (dialog)  Indices=1  OutputSizes=1
  If Action Subsystem1 : Subsystem  TreatAsAtomicUnit=on
  If Action Subsystem2 : Subsystem  TreatAsAtomicUnit=on
  If Action Subsystem3 : Subsystem  TreatAsAtomicUnit=on
  If Action Subsystem4 : Subsystem  TreatAsAtomicUnit=on
  If Action Subsystem5 : Subsystem  TreatAsAtomicUnit=on
  If Action Subsystem6 : Subsystem  TreatAsAtomicUnit=on
  If1 : If  ElseIfExpressions=u1 == 0
  If2 : If  ElseIfExpressions=u1 == 0
  wires:
  If2/1 -> If Action Subsystem4/Action
  Data Store Read8/1 -> If2/1
  If2/3 -> If Action Subsystem3/Action
  If2/2 -> If Action Subsystem1/Action
  If1/3 -> If Action Subsystem5/Action
  Data Store Read1/1 -> If1/1
  If1/1 -> If Action Subsystem6/Action
  If1/2 -> If Action Subsystem2/Action

== system Medium_Self_Balance_Vehicle/Function-Call Subsystem/Subsystem/If Action Subsystem ==
  Action Port : ActionPort  ActionPortLabel=if { }
  Constant1 : Constant  Value=0
  Data Store Write : DataStoreWrite  DataStoreName=LEDflash  IndexOptions=Index vector (dialog)  Indices=1  OutputSizes=1
  GPIO_Write : GPIO_Lib/GPIO_Write  Port_name=GPIOA  Pin0=off  Toggle_Pin0=off  Pin1=off  Toggle_Pin1=off  Pin2=off  Toggle_Pin2=off  Pin3=off  Toggle_Pin3=off  Pin4=on  Toggle_Pin4=on  Pin5=off  Toggle_Pin5=off  Pin6=off  Toggle_Pin6=off  Pin7=off  Toggle_Pin7=off  Pin8=off  Toggle_Pin8=off  Pin9=off  Toggle_Pin9=off  Pin10=off  Toggle_Pin10=off  Pin11=off  Toggle_Pin11=off  Pin12=off  Toggle_Pin12=off  Pin13=off  Toggle_Pin13=off  Pin14=off  Toggle_Pin14=off  Pin15=off  Toggle_Pin15=off  PinList="GPIOA4  15GPIOB3   4   5   8   9  12  13  14  15"
      settings: SourceProductName=Target Support Package - STM32 Adapter
  wires:
  Constant1/1 -> Data Store Write/1

== system Medium_Self_Balance_Vehicle/Function-Call Subsystem/Subsystem10/For Iterator Subsystem1 ==
  In1 : Inport
  Add : Sum
  For Iterator : ForIterator  ResetStates=reset  IterationLimit=10  ShowIterationPort=off
  Unit Delay : UnitDelay  SampleTime=-1  HasFrameUpgradeWarning=on
  Out1 : Outport  VectorParamsAs1DForOutWhenUnconnected=off
  wires:
  Add/1 -> Unit Delay/1, Out1/1
  Unit Delay/1 -> Add/2
  In1/1 -> Add/1

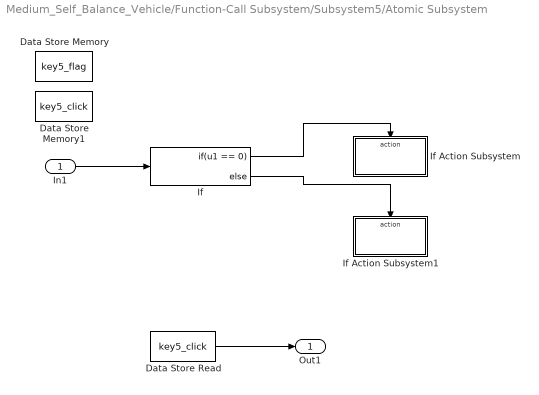
== system Medium_Self_Balance_Vehicle/Function-Call Subsystem/Subsystem5/Atomic Subsystem ==
  In1 : Inport
  Data Store Memory : DataStoreMemory  DataStoreName=key5_flag  ReadBeforeWriteMsg=warning  WriteAfterWriteMsg=warning  WriteAfterReadMsg=warning  ShowAdditionalParam=off  OutDataTypeStr=int16
  Data Store Memory1 : DataStoreMemory  DataStoreName=key5_click  ReadBeforeWriteMsg=warning  WriteAfterWriteMsg=warning  WriteAfterReadMsg=warning  ShowAdditionalParam=off  OutDataTypeStr=int16
  Data Store Read : DataStoreRead  Priority=5  DataStoreName=key5_click  IndexOptions=Index vector (dialog)  Indices=1  OutputSizes=1
  If : If  Priority=0  IfExpression=u1 == 0
  If Action Subsystem : Subsystem  TreatAsAtomicUnit=on
  If Action Subsystem1 : Subsystem  TreatAsAtomicUnit=on
  Out1 : Outport  OutDataTypeStr=int16  VectorParamsAs1DForOutWhenUnconnected=off
  wires:
  In1/1 -> If/1
  If/1 -> If Action Subsystem/Action
  If/2 -> If Action Subsystem1/Action
  Data Store Read/1 -> Out1/1

== system Medium_Self_Balance_Vehicle/Function-Call Subsystem/Subsystem5/If Action Subsystem ==
  Action Port : ActionPort  ActionPortLabel=if { }
  Data Store Read1 : DataStoreRead  DataStoreName=Flagstop  IndexOptions=Index vector (dialog)  Indices=1  OutputSizes=1
  Data Store Write1 : DataStoreWrite  DataStoreName=Flagstop  IndexOptions=Index vector (dialog)  Indices=1  OutputSizes=1
  Logical Operator : Logic  Operator=NOT  AllPortsSameDT=off  OutDataTypeStr=boolean
  wires:
  Logical Operator/1 -> Data Store Write1/1
  Data Store Read1/1 -> Logical Operator/1

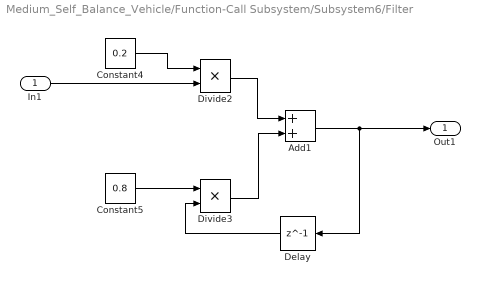
== system Medium_Self_Balance_Vehicle/Function-Call Subsystem/Subsystem6/Filter ==
  In1 : Inport
  Add1 : Sum
  Constant4 : Constant  Value=0.2
  Constant5 : Constant  Value=0.8
  Delay : Delay  DelayLength=1  InitialCondition=0
  Divide2 : Product  Inputs=**
  Divide3 : Product  Inputs=**
  Out1 : Outport  VectorParamsAs1DForOutWhenUnconnected=off
  wires:
  Divide2/1 -> Add1/1
  Constant4/1 -> Divide2/1
  Delay/1 -> Divide3/2
  Divide3/1 -> Add1/2
  In1/1 -> Divide2/2
  Constant5/1 -> Divide3/1
  Add1/1 -> Out1/1, Delay/1

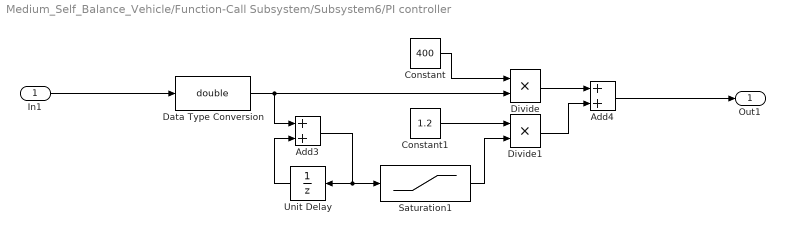
== system Medium_Self_Balance_Vehicle/Function-Call Subsystem/Subsystem6/PI controller ==
  In1 : Inport
  Add3 : Sum  Priority=2
  Add4 : Sum  Priority=2
  Constant : Constant  Value=400  OutDataTypeStr=double
  Constant1 : Constant  Value=1.2  OutDataTypeStr=double
  Data Type Conversion : DataTypeConversion  OutDataTypeStr=double
  Divide : Product  Inputs=**
  Divide1 : Product  Inputs=**
  Saturation1 : Saturate  UpperLimit=10000  LowerLimit=-10000
  Unit Delay : UnitDelay  SampleTime=-1  HasFrameUpgradeWarning=on
  Out1 : Outport  VectorParamsAs1DForOutWhenUnconnected=off
  wires:
  Saturation1/1 -> Divide1/2
  In1/1 -> Data Type Conversion/1
  Add3/1 -> Saturation1/1, Unit Delay/1
  Constant1/1 -> Divide1/1
  Divide1/1 -> Add4/2
  Data Type Conversion/1 -> Add3/1, Divide/2
  Divide/1 -> Add4/1
  Add4/1 -> Out1/1
  Unit Delay/1 -> Add3/2
  Constant/1 -> Divide/1

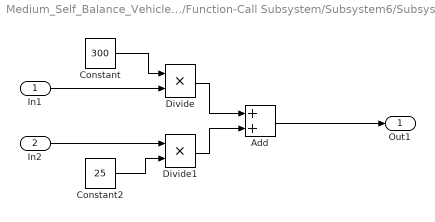
== system Medium_Self_Balance_Vehicle/Function-Call Subsystem/Subsystem6/Subsystem ==
  In1 : Inport
  In2 : Inport  Port=2
  Add : Sum
  Constant : Constant  Value=300
  Constant2 : Constant  Value=25
  Divide : Product  Inputs=**
  Divide1 : Product  Inputs=**
  Out1 : Outport  VectorParamsAs1DForOutWhenUnconnected=off
  wires:
  Divide1/1 -> Add/2
  Constant/1 -> Divide/1
  Constant2/1 -> Divide1/2
  Add/1 -> Out1/1
  Divide/1 -> Add/1
  In1/1 -> Divide/2
  In2/1 -> Divide1/1

== system Medium_Self_Balance_Vehicle/Function-Call Subsystem/Subsystem6/Subsystem1 ==
  In1 : Inport
  In2 : Inport  Port=2
  Add : Sum
  Constant : Constant  Value=10
  Constant2 : Constant  Value=-5
  Divide : Product  Inputs=**
  Divide1 : Product  Inputs=**
  Out1 : Outport  VectorParamsAs1DForOutWhenUnconnected=off
  wires:
  Divide1/1 -> Add/2
  Constant/1 -> Divide/1
  Constant2/1 -> Divide1/2
  Add/1 -> Out1/1
  Divide/1 -> Add/1
  In1/1 -> Divide/2
  In2/1 -> Divide1/1

== system Medium_Self_Balance_Vehicle/Function-Call Subsystem/Subsystem7/If Action Subsystem ==
  Action Port : ActionPort  ActionPortLabel=if { }
  Constant : Constant  OutDataTypeStr=boolean
  Data Store Write1 : DataStoreWrite  DataStoreName=Flagstop  IndexOptions=Index vector (dialog)  Indices=1  OutputSizes=1
  wires:
  Constant/1 -> Data Store Write1/1

== system Medium_Self_Balance_Vehicle/Function-Call Subsystem/Subsystem7/If Action Subsystem1 ==
  Action Port : ActionPort  ActionPortLabel=if { }
  Constant : Constant  OutDataTypeStr=boolean
  Data Store Write1 : DataStoreWrite  DataStoreName=Flagstop  IndexOptions=Index vector (dialog)  Indices=1  OutputSizes=1
  wires:
  Constant/1 -> Data Store Write1/1

== system Medium_Self_Balance_Vehicle/Function-Call Subsystem/Subsystem7/If Action Subsystem2 ==
  Action Port : ActionPort  ActionPortLabel=if { }
  Constant : Constant  Value=0  OutDataTypeStr=double
  Constant1 : Constant  Value=0  OutDataTypeStr=double
  Data Store Write1 : DataStoreWrite  DataStoreName=MotorA  IndexOptions=Index vector (dialog)  Indices=1  OutputSizes=1
  Data Store Write2 : DataStoreWrite  DataStoreName=MotorB  IndexOptions=Index vector (dialog)  Indices=1  OutputSizes=1
  wires:
  Constant/1 -> Data Store Write1/1
  Constant1/1 -> Data Store Write2/1

== system Medium_Self_Balance_Vehicle/Function-Call Subsystem/Subsystem9/If Action Subsystem1 ==
  Action Port : ActionPort  ActionPortLabel=elseif { }
  Constant : Constant  Value=0
  Constant1 : Constant  Value=0
  Data Store Read1 : DataStoreRead  DataStoreName=motoa  IndexOptions=Index vector (dialog)  Indices=1  OutputSizes=1
  GPIO_Write1 : GPIO_Lib/GPIO_Write  Port_name=GPIOB  Pin0=off  Toggle_Pin0=off  Pin1=off  Toggle_Pin1=off  Pin2=off  Toggle_Pin2=off  Pin3=off  Toggle_Pin3=off  Pin4=off  Toggle_Pin4=off  Pin5=off  Toggle_Pin5=off  Pin6=off  Toggle_Pin6=off  Pin7=off  Toggle_Pin7=off  Pin8=off  Toggle_Pin8=off  Pin9=off  Toggle_Pin9=off  Pin10=off  Toggle_Pin10=off  Pin11=off  Toggle_Pin11=off  Pin12=off  Toggle_Pin12=off  Pin13=off  Toggle_Pin13=off  Pin14=on  Toggle_Pin14=off  Pin15=on  Toggle_Pin15=off  PinList="GPIOA4  15GPIOB3   4   5   8   9  12  13  14  15"
      settings: SourceProductName=Target Support Package - STM32 Adapter
  Timers : TIMERS_Lib/Timers  currentTIM=TIM1  TIM_Name=TIM1  sysUsingTimer=off  TIM_APBClock=72000000  TIM_Set_Clk=off  TIM_Prescaler=0  TIM_Clock=72000000.00  Variable_frequency=off  TIM_Set_OutFreq=off  TIM_ARR=7200  Output_frequency=10000.00  Repetition_counter=0  TIM_Mode=Up  TIM_DMA=none  TIM_IRQ=off  TIM_IRQ_ONLY=off  TIM_UP=off  TIM_TRG=off  TIM_COM=off  TIM_BRK=off  NbTIM=4  CH1_enable=on  CH1N_enable=off  CH1_type=Output_PWM  CH1_DMA=off  CH1_int=off  CH1_edge=Rising  CH1_div=1  CH1_variable_duty=on  CH1_set_pulse=off  CH1_output_duty=0.00  CH1_pulse=0  CH2_enable=off  CH2N_enable=off  CH2_type=Unknown  CH2_DMA=off  CH2_int=off  CH2_edge=Rising  CH2_div=1  CH2_variable_duty=off  CH2_set_pulse=off  CH2_output_duty=0.00  CH2_pulse=0  CH3_enable=off  CH3N_enable=off  CH3_type=Unknown  CH3_DMA=off  CH3_int=off  CH3_edge=Rising  CH3_div=1  CH3_variable_duty=off  CH3_set_pulse=off  CH3_output_duty=0.00  CH3_pulse=0  CH4_enable=on  CH4N_enable=off  CH4_type=Output_PWM  CH4_DMA=off  CH4_int=off  CH4_edge=Rising  CH4_div=1  CH4_variable_duty=off  CH4_set_pulse=off  CH4_output_duty=0.00  CH4_pulse=0
      settings: SourceProductName=Target Support Package - STM32 Adapter
  wires:
  Constant1/1 -> GPIO_Write1/1
  Data Store Read1/1 -> Timers/1
  Constant/1 -> GPIO_Write1/2

== system Medium_Self_Balance_Vehicle/Function-Call Subsystem/Subsystem9/If Action Subsystem2 ==
  Action Port : ActionPort  ActionPortLabel=elseif { }
  Constant : Constant  Value=0
  Constant1 : Constant  Value=0
  Data Store Read1 : DataStoreRead  DataStoreName=motob  IndexOptions=Index vector (dialog)  Indices=1  OutputSizes=1
  GPIO_Write1 : GPIO_Lib/GPIO_Write  Port_name=GPIOB  Pin0=off  Toggle_Pin0=off  Pin1=off  Toggle_Pin1=off  Pin2=off  Toggle_Pin2=off  Pin3=off  Toggle_Pin3=off  Pin4=off  Toggle_Pin4=off  Pin5=off  Toggle_Pin5=off  Pin6=off  Toggle_Pin6=off  Pin7=off  Toggle_Pin7=off  Pin8=off  Toggle_Pin8=off  Pin9=off  Toggle_Pin9=off  Pin10=off  Toggle_Pin10=off  Pin11=off  Toggle_Pin11=off  Pin12=on  Toggle_Pin12=off  Pin13=on  Toggle_Pin13=off  Pin14=off  Toggle_Pin14=off  Pin15=off  Toggle_Pin15=off  PinList="GPIOA4  15GPIOB3   4   5   8   9  12  13  14  15"
      settings: SourceProductName=Target Support Package - STM32 Adapter
  Timers : TIMERS_Lib/Timers  currentTIM=TIM1  TIM_Name=TIM1  sysUsingTimer=off  TIM_APBClock=72000000  TIM_Set_Clk=off  TIM_Prescaler=0  TIM_Clock=72000000.00  Variable_frequency=off  TIM_Set_OutFreq=off  TIM_ARR=7200  Output_frequency=10000.00  Repetition_counter=0  TIM_Mode=Up  TIM_DMA=none  TIM_IRQ=off  TIM_IRQ_ONLY=off  TIM_UP=off  TIM_TRG=off  TIM_COM=off  TIM_BRK=off  NbTIM=4  CH1_enable=on  CH1N_enable=off  CH1_type=Output_PWM  CH1_DMA=off  CH1_int=off  CH1_edge=Rising  CH1_div=1  CH1_variable_duty=off  CH1_set_pulse=off  CH1_output_duty=0.00  CH1_pulse=0  CH2_enable=off  CH2N_enable=off  CH2_type=Unknown  CH2_DMA=off  CH2_int=off  CH2_edge=Rising  CH2_div=1  CH2_variable_duty=off  CH2_set_pulse=off  CH2_output_duty=0.00  CH2_pulse=0  CH3_enable=off  CH3N_enable=off  CH3_type=Unknown  CH3_DMA=off  CH3_int=off  CH3_edge=Rising  CH3_div=1  CH3_variable_duty=off  CH3_set_pulse=off  CH3_output_duty=0.00  CH3_pulse=0  CH4_enable=on  CH4N_enable=off  CH4_type=Output_PWM  CH4_DMA=off  CH4_int=off  CH4_edge=Rising  CH4_div=1  CH4_variable_duty=on  CH4_set_pulse=off  CH4_output_duty=0.00  CH4_pulse=0
      settings: SourceProductName=Target Support Package - STM32 Adapter
  wires:
  Constant1/1 -> GPIO_Write1/1
  Data Store Read1/1 -> Timers/1
  Constant/1 -> GPIO_Write1/2

== system Medium_Self_Balance_Vehicle/Function-Call Subsystem/Subsystem9/If Action Subsystem3 ==
  Action Port : ActionPort  ActionPortLabel=else { }
  Constant1 : Constant  Value=-1  OutDataTypeStr=int16
  Constant3 : Constant
  Constant4 : Constant  Value=0
  Data Store Read1 : DataStoreRead  DataStoreName=motoa  IndexOptions=Index vector (dialog)  Indices=1  OutputSizes=1
  Divide : Product  Inputs=**
  GPIO_Write3 : GPIO_Lib/GPIO_Write  Port_name=GPIOB  Pin0=off  Toggle_Pin0=off  Pin1=off  Toggle_Pin1=off  Pin2=off  Toggle_Pin2=off  Pin3=off  Toggle_Pin3=off  Pin4=off  Toggle_Pin4=off  Pin5=off  Toggle_Pin5=off  Pin6=off  Toggle_Pin6=off  Pin7=off  Toggle_Pin7=off  Pin8=off  Toggle_Pin8=off  Pin9=off  Toggle_Pin9=off  Pin10=off  Toggle_Pin10=off  Pin11=off  Toggle_Pin11=off  Pin12=off  Toggle_Pin12=off  Pin13=off  Toggle_Pin13=off  Pin14=on  Toggle_Pin14=off  Pin15=on  Toggle_Pin15=off  PinList="GPIOA4  15GPIOB3   4   5   8   9  12  13  14  15"
      settings: SourceProductName=Target Support Package - STM32 Adapter
  Timers : TIMERS_Lib/Timers  currentTIM=TIM1  TIM_Name=TIM1  sysUsingTimer=off  TIM_APBClock=72000000  TIM_Set_Clk=off  TIM_Prescaler=0  TIM_Clock=72000000.00  Variable_frequency=off  TIM_Set_OutFreq=off  TIM_ARR=7200  Output_frequency=10000.00  Repetition_counter=0  TIM_Mode=Up  TIM_DMA=none  TIM_IRQ=off  TIM_IRQ_ONLY=off  TIM_UP=off  TIM_TRG=off  TIM_COM=off  TIM_BRK=off  NbTIM=4  CH1_enable=on  CH1N_enable=off  CH1_type=Output_PWM  CH1_DMA=off  CH1_int=off  CH1_edge=Rising  CH1_div=1  CH1_variable_duty=on  CH1_set_pulse=off  CH1_output_duty=0.00  CH1_pulse=0  CH2_enable=off  CH2N_enable=off  CH2_type=Unknown  CH2_DMA=off  CH2_int=off  CH2_edge=Rising  CH2_div=1  CH2_variable_duty=off  CH2_set_pulse=off  CH2_output_duty=0.00  CH2_pulse=0  CH3_enable=off  CH3N_enable=off  CH3_type=Unknown  CH3_DMA=off  CH3_int=off  CH3_edge=Rising  CH3_div=1  CH3_variable_duty=off  CH3_set_pulse=off  CH3_output_duty=0.00  CH3_pulse=0  CH4_enable=on  CH4N_enable=off  CH4_type=Output_PWM  CH4_DMA=off  CH4_int=off  CH4_edge=Rising  CH4_div=1  CH4_variable_duty=off  CH4_set_pulse=off  CH4_output_duty=0.00  CH4_pulse=0
      settings: SourceProductName=Target Support Package - STM32 Adapter
  wires:
  Constant1/1 -> Divide/2
  Data Store Read1/1 -> Divide/1
  Constant4/1 -> GPIO_Write3/1
  Constant3/1 -> GPIO_Write3/2
  Divide/1 -> Timers/1

== system Medium_Self_Balance_Vehicle/Function-Call Subsystem/Subsystem9/If Action Subsystem4 ==
  Action Port : ActionPort  ActionPortLabel=if { }
  Constant : Constant  Value=0
  Constant1 : Constant
  Data Store Read1 : DataStoreRead  DataStoreName=motoa  IndexOptions=Index vector (dialog)  Indices=1  OutputSizes=1
  GPIO_Write1 : GPIO_Lib/GPIO_Write  Port_name=GPIOB  Pin0=off  Toggle_Pin0=off  Pin1=off  Toggle_Pin1=off  Pin2=off  Toggle_Pin2=off  Pin3=off  Toggle_Pin3=off  Pin4=off  Toggle_Pin4=off  Pin5=off  Toggle_Pin5=off  Pin6=off  Toggle_Pin6=off  Pin7=off  Toggle_Pin7=off  Pin8=off  Toggle_Pin8=off  Pin9=off  Toggle_Pin9=off  Pin10=off  Toggle_Pin10=off  Pin11=off  Toggle_Pin11=off  Pin12=off  Toggle_Pin12=off  Pin13=off  Toggle_Pin13=off  Pin14=on  Toggle_Pin14=off  Pin15=on  Toggle_Pin15=off  PinList="GPIOA4  15GPIOB3   4   5   8   9  12  13  14  15"
      settings: SourceProductName=Target Support Package - STM32 Adapter
  Timers : TIMERS_Lib/Timers  currentTIM=TIM1  TIM_Name=TIM1  sysUsingTimer=off  TIM_APBClock=72000000  TIM_Set_Clk=off  TIM_Prescaler=0  TIM_Clock=72000000.00  Variable_frequency=off  TIM_Set_OutFreq=off  TIM_ARR=7199  Output_frequency=10001.39  Repetition_counter=0  TIM_Mode=Up  TIM_DMA=none  TIM_IRQ=off  TIM_IRQ_ONLY=off  TIM_UP=off  TIM_TRG=off  TIM_COM=off  TIM_BRK=off  NbTIM=4  CH1_enable=on  CH1N_enable=off  CH1_type=Output_PWM  CH1_DMA=off  CH1_int=off  CH1_edge=Rising  CH1_div=1  CH1_variable_duty=on  CH1_set_pulse=off  CH1_output_duty=0.00  CH1_pulse=0  CH2_enable=off  CH2N_enable=off  CH2_type=Unknown  CH2_DMA=off  CH2_int=off  CH2_edge=Rising  CH2_div=1  CH2_variable_duty=off  CH2_set_pulse=off  CH2_output_duty=0.00  CH2_pulse=0  CH3_enable=off  CH3N_enable=off  CH3_type=Unknown  CH3_DMA=off  CH3_int=off  CH3_edge=Rising  CH3_div=1  CH3_variable_duty=off  CH3_set_pulse=off  CH3_output_duty=0.00  CH3_pulse=0  CH4_enable=on  CH4N_enable=off  CH4_type=Output_PWM  CH4_DMA=off  CH4_int=off  CH4_edge=Rising  CH4_div=1  CH4_variable_duty=off  CH4_set_pulse=off  CH4_output_duty=0.00  CH4_pulse=0
      settings: SourceProductName=Target Support Package - STM32 Adapter
  wires:
  Constant/1 -> GPIO_Write1/2
  Constant1/1 -> GPIO_Write1/1
  Data Store Read1/1 -> Timers/1
